simulink model "triad_estimator_error_test"  (R2018b)
settings: Solver=VariableStepAuto  StartTime=0.0  StopTime=1.0  RelTol=1e-3
values from neighbouring files (symbols this model uses):
  dcm_true = rot(eul(1),'x') * rot(eul(2),'y') * rot(eul(3),'z')    [triad_estimator_error_test_init.m]
  vec_body_1 = dcm_true * vec_eci_1    [triad_estimator_error_test_init.m]
  vec_body_2 = dcm_true * vec_eci_2    [triad_estimator_error_test_init.m]
  vec_eci_1 = vec_eci_1./norm(vec_eci_1)    [triad_estimator_error_test_init.m]
  vec_eci_2 = rotk * vec_eci_1    [triad_estimator_error_test_init.m]
libraries: sharedtransform x1, Triad_lib x1, quat_degerr_lib x1
settings Model: Creator=Taylor  LastModifiedBy=Taylor

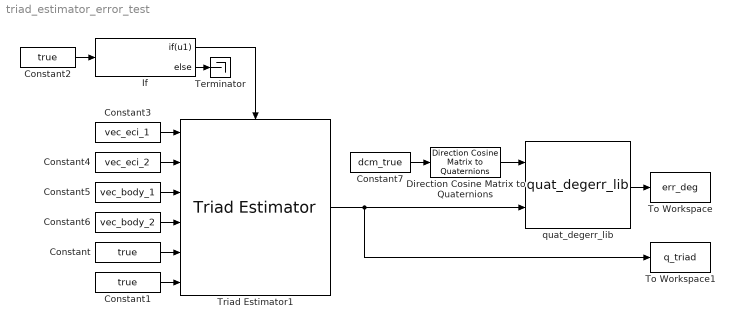
== system triad_estimator_error_test ==
  Constant : Constant  Value=true
  Constant1 : Constant  Value=true
  Constant2 : Constant  Value=true
  Constant3 : Constant  Value=vec_eci_1
  Constant4 : Constant  Value=vec_eci_2
  Constant5 : Constant  Value=vec_body_1
  Constant6 : Constant  Value=vec_body_2
  Constant7 : Constant  Value=dcm_true
  Direction Cosine Matrix to Quaternions : sharedtransform/Direction Cosine Matrix  to Quaternions  aMode=0  action=None  tolerance=eps(2)
      settings: SourceProductName=Aerospace Blockset  SourceProductBaseCode=AE
  If : If  IfExpression=u1
  Terminator : Terminator
  To Workspace : ToWorkspace  VariableName=err_deg  SampleTime=-1
      settings: MaxDataPoints=1
  To Workspace1 : ToWorkspace  VariableName=q_triad  SampleTime=-1
      settings: MaxDataPoints=1
  Triad Estimator1 : Triad_lib/Triad Estimator  SystemSampleTime=-1
  quat_degerr_lib : quat_degerr_lib/quat_degerr_lib  SystemSampleTime=-1
  wires:
  Constant/1 -> Triad Estimator1/5
  Constant1/1 -> Triad Estimator1/6
  Constant2/1 -> If/1
  If/1 -> Triad Estimator1/Action
  If/2 -> Terminator/1
  Constant3/1 -> Triad Estimator1/1
  Constant4/1 -> Triad Estimator1/2
  Constant5/1 -> Triad Estimator1/3
  Constant6/1 -> Triad Estimator1/4
  Constant7/1 -> Direction Cosine Matrix to Quaternions/1
  quat_degerr_lib/1 -> To Workspace/1
  Triad Estimator1/1 -> quat_degerr_lib/2, To Workspace1/1
  Direction Cosine Matrix to Quaternions/1 -> quat_degerr_lib/1
